simulink model "model"  (R2021b)
settings: Solver=VariableStepAuto  StartTime=0.0  StopTime=10.0  RelTol=1e-3
libraries: simulink x1
settings Model: SimulationMode=accelerator  Creator=O1  LastModifiedBy=wangzixuan

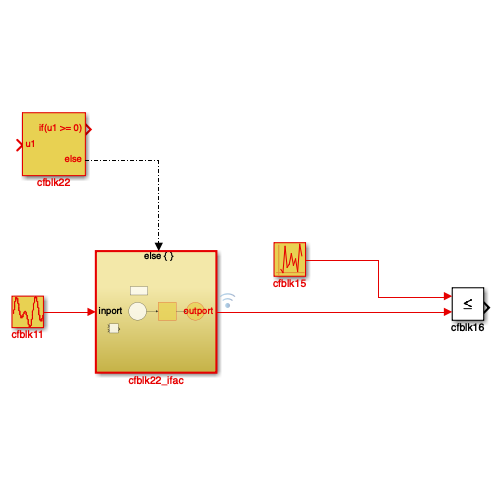
[thumbnail: Simulink's stored preview of the top-level diagram]
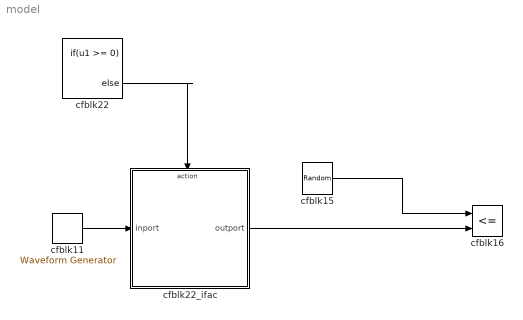
== system model ==
  cfblk11 : simulink/Sources/Waveform Generator  OutMin=[]  OutMax=[]  OutDataTypeStr=double  SelectedSignal=1  BlockNames=MultiportSwitch_e3df3653d217406  SampleTime=0.1
  cfblk15 : UniformRandomNumber  SampleTime=0.1
  cfblk16 : RelationalOperator  Operator=<=  OutDataTypeStr=boolean  RndMeth=Simplest
  cfblk22 : If  IfExpression=u1 >= 0  SampleTime=1
  cfblk22_ifac : Subsystem  TreatAsAtomicUnit=on
  wires:
  cfblk11/1 -> cfblk22_ifac/1(inport)
  cfblk22/2 -> cfblk22_ifac/Action
  cfblk15/1 -> cfblk16/1
  cfblk22_ifac/1(outport) -> cfblk16/2

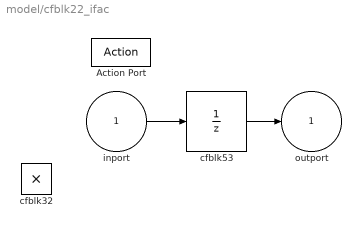
== system model/cfblk22_ifac ==
  inport : Inport
  Action Port : ActionPort  ActionPortLabel=else
  cfblk32 : Product
  cfblk53 : UnitDelay  SampleTime=-1  HasFrameUpgradeWarning=on
  outport : Outport
  wires:
  inport/1 -> cfblk53/1
  cfblk53/1 -> outport/1
